simulink model "fcs_lab_05_model_03"  (R2014b)
settings: Solver=ode45  StartTime=0.0  StopTime=500  RelTol=1e-3
values from neighbouring files (symbols this model uses):
  C = 10    [fcs_lab_05_model_02_test.m]    (also in fcs_lab_05_model_03_test.m)
  e = 60    [fcs_lab_05_model_02_test.m]    (also in fcs_lab_05_model_03_test.m)
  L1 = 1    [fcs_lab_05_model_03_test.m]
  L2 = 1    [fcs_lab_05_model_03_test.m]
  R1 = 10    [fcs_lab_05_model_03_test.m]
  R2 = 10    [fcs_lab_05_model_03_test.m]
settings Model: Creator=Mashkoor Ahmed  LastModifiedBy=Mashkoor Ahmed

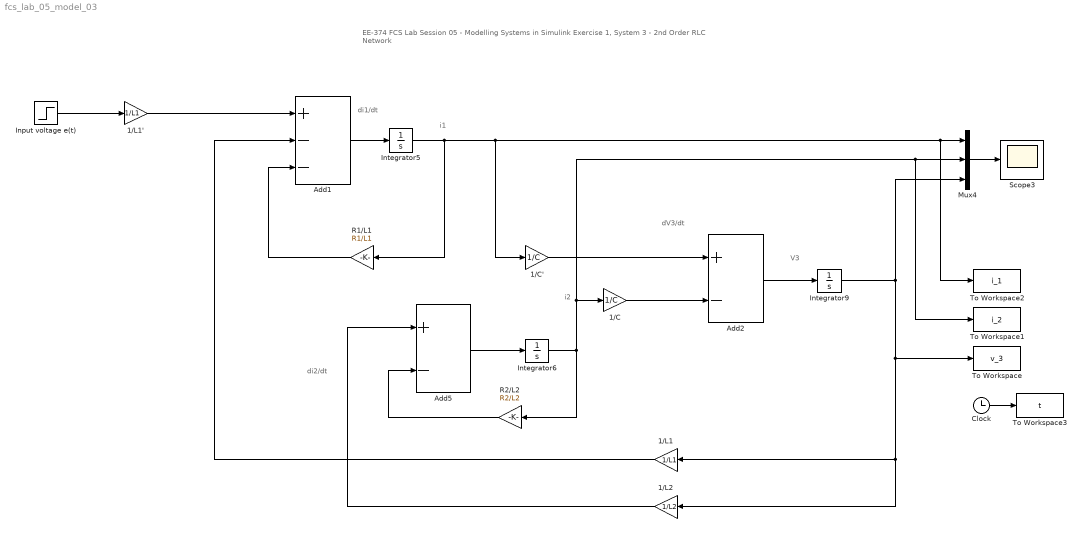
== system fcs_lab_05_model_03 ==
  note: EE-374 FCS Lab Session 05 - Modelling Systems in Simulink
      | Exercise 1, System 3 - 2nd Order RLC Network
  note: di1/dt
  note: i1
  note: i2
  note: V3
  note: dV3/dt
  note: di2/dt
  1/C : Gain  Gain=1/C
  1/C' : Gain  Gain=1/C
  1/L1 : Gain  Gain=1/L1
  "1/L1' " : Gain  Gain=1/L1
  1/L2 : Gain  Gain=1/L2
  Add1 : Sum  Inputs=+--
  Add2 : Sum  Inputs=+-
  Add5 : Sum  Inputs=+-
  Clock : Clock
  Input voltage e(t) : Step  Time=0  After=e  SampleTime=0
  Integrator5 : Integrator
  Integrator6 : Integrator
  Integrator9 : Integrator
  Mux4 : Mux  Inputs=3
  R1/L1 : Gain  Gain=R1/L1
  R2/L2 : Gain  Gain=R2/L2
  Scope3 : Scope
      settings: YMin=-3.68036  YMax=33.12327  SaveName=ScopeData3
  To Workspace : ToWorkspace  VariableName=v_3  SampleTime=-1
  To Workspace1 : ToWorkspace  VariableName=i_2  SampleTime=-1
  To Workspace2 : ToWorkspace  VariableName=i_1  SampleTime=-1
  To Workspace3 : ToWorkspace  VariableName=t  SampleTime=-1
  wires:
  Add1/1 -> Integrator5/1
  Integrator5/1 -> 1/C'/1, To Workspace2/1, Mux4/1, R1/L1/1
  Mux4/1 -> Scope3/1
  "1/L1' "/1 -> Add1/1
  Input voltage e(t)/1 -> "1/L1' "/1
  Add5/1 -> Integrator6/1
  Integrator6/1 -> To Workspace1/1, Mux4/2, 1/C/1, R2/L2/1
  R2/L2/1 -> Add5/2
  Add2/1 -> Integrator9/1
  1/C'/1 -> Add2/1
  1/C/1 -> Add2/2
  Integrator9/1 -> Mux4/3, 1/L2/1, 1/L1/1, To Workspace/1
  1/L2/1 -> Add5/1
  1/L1/1 -> Add1/2
  R1/L1/1 -> Add1/3
  Clock/1 -> To Workspace3/1
